simulink model "model_VS_PSH"  (R2020b)
settings: Solver=ode1  StartTime=0.0  StopTime=60  RelTol=1e-3
InitFcn:
  | xInitial = init_power_wind_dfig_det;
  | %Ts=5e-6;
values from neighbouring files (symbols this model uses):
  Cap_DClink = 20000e-6    (= 0.02)    [MAIN_VS_PSH.m]
  Efficiency = 0.9    [MAIN_VS_PSH.m]
  Fnom = 60    [MAIN_VS_PSH.m]
  H = 2.7    [MAIN_VS_PSH.m]
  Initial_Head = 1    [MAIN_VS_PSH.m]
  Initial_SOC = 0.8    [MAIN_VS_PSH.m]
  kmVdc = 20e3    (= 20000)    [MAIN_VS_PSH.m]
  Kp = 1    [MAIN_VS_PSH.m]
  kp_pll = 0.236583    [MAIN_T_PSH_IEEE39.m]    (also in MAIN_VS_PSH.m)
  Kpg = 1.3466e-5    (= 1.3466e-05)    [MAIN_VS_PSH.m]
  Kpr = 4.559e-5    (= 4.559e-05)    [MAIN_VS_PSH.m]
  Kvp = 6.1584    [MAIN_VS_PSH.m]
  Lm = Lb*Lmpu    [MAIN_VS_PSH.m]
  Lph = 3e-4    (= 0.0003)    [MAIN_VS_PSH.m]
  Lr = Lb*Lrpu    [MAIN_VS_PSH.m]
  Lrleakpu = 0.11    [MAIN_VS_PSH.m]
  Ls = Lb*Lspu    [MAIN_VS_PSH.m]
  Lsleakpu = 0.102    [MAIN_VS_PSH.m]
  Max_discharge_hrs = 10    [MAIN_VS_PSH.m]
  Mode = 0    [MAIN_FS_PSH_IEEE39.m]    (also in MAIN_VS_PSH.m = 1; plots_FS_PSH_IEEE39.m = 1; plots_VS_PSH.m = 1)
  Pnom = Srated*1e6    (= 300000000)    [MAIN_VS_PSH.m]
  Pref = 0.9    [MAIN_T_PSH_IEEE39.m]    (also in MAIN_VS_PSH.m = 1)
  QnL = 0    [MAIN_VS_PSH.m]
  Qref = 0    [MAIN_VS_PSH.m]
  Rrpu = 0.00607    [MAIN_VS_PSH.m]
  Rspu = 0.0054    [MAIN_VS_PSH.m]
  sigma = 1- Lmpu*Lmpu/(Lrpu^2)    (= 0.0485899542692)    [MAIN_VS_PSH.m]
  Srated = 300    [MAIN_VS_PSH.m]
  t_sw_off = 220    [MAIN_FS_PSH_IEEE39.m]    (also in MAIN_T_PSH_IEEE39.m; MAIN_VS_PSH.m = 45)
  t_sw_on = 130    [MAIN_FS_PSH_IEEE39.m]    (also in MAIN_T_PSH_IEEE39.m; MAIN_VS_PSH.m = 35)
  Ti = 0.01    [MAIN_VS_PSH.m]
  ti_pll = 0.0224242    [MAIN_T_PSH_IEEE39.m]    (also in MAIN_VS_PSH.m)
  Tig = 59.0944    [MAIN_VS_PSH.m]
  Tir = 197.953    [MAIN_VS_PSH.m]
  Ts = 25e-6    (= 2.5e-05)    [MAIN_FS_PSH_IEEE39.m]    (also in MAIN_T_PSH_IEEE39.m; MAIN_VS_PSH.m = 1e-07)
  TurnsRatio = 0.37912    [MAIN_VS_PSH.m]
  Tvi = 0.0013532    [MAIN_VS_PSH.m]
  V1 = sqrt(2)*Vnom_grid/sqrt(3)    [MAIN_VS_PSH.m]
  Vdc_ref = 40e3    (= 40000)    [MAIN_VS_PSH.m]
  Vnom_grid = 18e3    (= 18000)    [MAIN_VS_PSH.m]
  W1 = 2*pi*Fnom    (= 376.991118431)    [MAIN_VS_PSH.m]
  Xph = Lph*W1    (= 0.113097335529)    [MAIN_VS_PSH.m]
undefined symbols (not defined in the file or in its folder): magnitude
libraries: powerlib x49, powerlib_meascontrol x21, pid_lib x10, simulink_extras x4, simulink x1
(part 3 of 3)

== system model_VS_PSH/Subsystem2/Subsystem5/Measurement and Transformation/Subsystem ==
  Vabc : Inport
  Constant : Constant  Value=2*pi*60
  Demux : Demux  Outputs=3
  Gain : Gain  Gain=1/(2*pi)
  Integrator : Integrator
  MATLAB Function1 : MATLAB Function  TreatAsAtomicUnit=on
  PID Controller : pid_lib/PID Controller  Controller=PI  Form=Parallel  TimeDomain=Continuous-time  UseExternalTs=off  SampleTime=-1  IntegratorMethod=Forward Euler  FilterMethod=Forward Euler  ControllerParametersSource=internal  P=kp_pll  I=kp_pll/ti_pll  D=0  UseFilter=on  N=100  TunerSelectOption=Transfer Function Based (PID Tuner App)  InitialConditionSource=internal  InitialConditionForIntegrator=0  InitialConditionForFilter=0  DifferentiatorICPrevScaledInput=0  ExternalReset=none  TrackingMode=off  Kt=1  LimitOutput=off  SatLimitsSource=internal  UpperSaturationLimit=inf  LowerSaturationLimit=-inf  LinearizeAsGain=on  AntiWindupMode=none  Kb=1  POutMin=[]  POutMax=[]  IOutMin=[]  IOutMax=[]  DOutMin=[]  DOutMax=[]  NOutMin=[]  NOutMax=[]  SumOutMin=[]  SumOutMax=[]  SaturationOutMin=[]  SaturationOutMax=[]  PParamMin=[]  PParamMax=[]  IParamMin=[]  IParamMax=[]  DParamMin=[]  DParamMax=[]  NParamMin=[]  NParamMax=[]  KbParamMin=[]  KbParamMax=[]  KtParamMin=[]  KtParamMax=[]  KbOutMin=[]  KbOutMax=[]  KtOutMin=[]  KtOutMax=[]  IntegratorOutMin=[]  IntegratorOutMax=[]  FilterOutMin=[]  FilterOutMax=[]  SumI1OutMin=[]  SumI1OutMax=[]  SumI2OutMin=[]  SumI2OutMax=[]  SumI3OutMin=[]  SumI3OutMax=[]  SumI4OutMin=[]  SumI4OutMax=[]  SumDOutMin=[]  SumDOutMax=[]  DifferentiatorOutMin=[]  DifferentiatorOutMax=[]  FilterDiffOutCoefMin=[]  FilterDiffOutCoefMax=[]  ReciprocalOutMin=[]  ReciprocalOutMax=[]  SumDenOutMin=[]  SumDenOutMax=[]  SumNumOutMin=[]  SumNumOutMax=[]  DivideOutMin=[]  DivideOutMax=[]  UdiffTsProdOutMin=[]  UdiffTsProdOutMax=[]  NTsProdOutMin=[]  NTsProdOutMax=[]  UintegralTsProdOutMin=[]  UintegralTsProdOutMax=[]  UngainTsProdOutMin=[]  UngainTsProdOutMax=[]  IntegratorContinuousStateAttributes=''  IntegratorStateMustResolveToSignalObject=off  IntegratorRTWStateStorageClass=Auto  FilterContinuousStateAttributes=''  FilterStateMustResolveToSignalObject=off  FilterRTWStateStorageClass=Auto  ParallelPVariant=InternalParameters  IdealPVariant=Disabled  IVariant=InternalParameters  DVariant=Disabled  IntegratorVariant=Continuous  SatVariant=Disabled  AWVariant=Passthrough  PCopyVariant=Disabled  TRVariant=Disabled  FdbkBlocksVariant=Forward  IdealPFdbkVariant=Disabled  SatFdbkVariant=Disabled  DerivativeFilterVariant=Disabled  NVariant=Disabled  NCopyVariant=Disabled_SignalSpec  FilterICVariant=Disabled  IntegratorICVariant=InternalICs  ExternalResetVariant=Disabled  TRSumVariant=Passthrough  SumFdbkVariant=Disabled  SumVariant=Sum_PI  TsampFilterVariant=InternalTs  TsampNgainVariant=Passthrough  TsampIntegralVariant=Passthrough  ExternalSaturationOutDataTypeStr=Inherit: Same as second input
  Scope2 : Scope
  Sum5 : Sum  Inputs=|++
  Terminator : Terminator
  Terminator1 : Terminator
  abc to dq0 : powerlib_meascontrol/Transformations/abc to dq0  Alignment=Aligned with phase A axis
  angle : Outport
  Freq_Hz : Outport  Port=2
  wires:
  Constant/1 -> Sum5/2
  PID Controller/1 -> Sum5/1
  Vabc/1 -> abc to dq0/1
  Demux/3 -> Terminator/1
  Demux/1 -> Terminator1/1
  Demux/2 -> PID Controller/1
  Sum5/1 -> Gain/1, Integrator/1
  Integrator/1 -> Scope2/1, MATLAB Function1/1(u)
  Gain/1 -> Freq_Hz/1
  MATLAB Function1/1(y) -> abc to dq0/2, angle/1
  abc to dq0/1 -> Demux/1

== system model_VS_PSH/Subsystem2/Subsystem5/Rotor-side Controls/Subsystem1 ==
  In : Inport
  Gain1 : Gain  Gain=1/Ti
  Gain2 : Gain  Gain=Kp
  Gain3 : Gain
  Integrator : Integrator
  Saturation : Saturate  UpperLimit=100e3  LowerLimit=-100e3
  Sum2 : Sum  Inputs=|++
  Sum3 : Sum  Inputs=-+|
  Sum7 : Sum  Inputs=|++
  Out : Outport
  wires:
  In/1 -> Sum7/1, Gain2/1
  Saturation/1 -> Sum3/2, Out/1
  Gain2/1 -> Sum2/1
  Sum2/1 -> Sum3/1, Saturation/1
  Sum3/1 -> Gain3/1
  Gain1/1 -> Integrator/1
  Integrator/1 -> Sum2/2
  Gain3/1 -> Sum7/2
  Sum7/1 -> Gain1/1

== system model_VS_PSH/Subsystem2/Subsystem5/Rotor-side Controls/Subsystem2 ==
  In : Inport
  Gain1 : Gain  Gain=1/Ti
  Gain2 : Gain  Gain=Kp
  Gain3 : Gain
  Integrator : Integrator
  Saturation : Saturate  UpperLimit=100e3  LowerLimit=-100e3
  Sum2 : Sum  Inputs=|++
  Sum3 : Sum  Inputs=-+|
  Sum7 : Sum  Inputs=|++
  Out : Outport
  wires:
  In/1 -> Sum7/1, Gain2/1
  Saturation/1 -> Sum3/2, Out/1
  Gain2/1 -> Sum2/1
  Sum2/1 -> Sum3/1, Saturation/1
  Sum3/1 -> Gain3/1
  Gain1/1 -> Integrator/1
  Integrator/1 -> Sum2/2
  Gain3/1 -> Sum7/2
  Sum7/1 -> Gain1/1

== system model_VS_PSH/Subsystem2/Subsystem5/Rotor-side Controls/Subsystem3 ==
  In : Inport
  Gain1 : Gain  Gain=1/Ti
  Gain2 : Gain  Gain=Kp
  Gain3 : Gain
  Integrator : Integrator
  Saturation : Saturate  UpperLimit=100e3  LowerLimit=-100e3
  Sum2 : Sum  Inputs=|++
  Sum3 : Sum  Inputs=-+|
  Sum7 : Sum  Inputs=|++
  Out : Outport
  wires:
  In/1 -> Sum7/1, Gain2/1
  Saturation/1 -> Sum3/2, Out/1
  Gain2/1 -> Sum2/1
  Sum2/1 -> Sum3/1, Saturation/1
  Sum3/1 -> Gain3/1
  Gain1/1 -> Integrator/1
  Integrator/1 -> Sum2/2
  Gain3/1 -> Sum7/2
  Sum7/1 -> Gain1/1

== system model_VS_PSH/Subsystem2/Subsystem5/Rotor-side Controls/Subsystem4 ==
  In : Inport
  Gain1 : Gain  Gain=1/Ti
  Gain2 : Gain  Gain=Kp
  Gain3 : Gain
  Integrator : Integrator
  Saturation : Saturate  UpperLimit=100e3  LowerLimit=-100e3
  Sum2 : Sum  Inputs=|++
  Sum3 : Sum  Inputs=-+|
  Sum7 : Sum  Inputs=|++
  Out : Outport
  wires:
  In/1 -> Sum7/1, Gain2/1
  Saturation/1 -> Sum3/2, Out/1
  Gain2/1 -> Sum2/1
  Sum2/1 -> Sum3/1, Saturation/1
  Sum3/1 -> Gain3/1
  Gain1/1 -> Integrator/1
  Integrator/1 -> Sum2/2
  Gain3/1 -> Sum7/2
  Sum7/1 -> Gain1/1

== matlab function model_VS_PSH/Subsystem2/Subsystem5/Measurement and Transformation/MATLAB Function2 ==
  data: u input; y output
function y = fcn(u)



if u>= 2*pi
    y = mod(u,2*pi);
elseif u <= 0
    y = 2*pi - mod(abs(u),2*pi);
else
    y = u;
end

== matlab function model_VS_PSH/Subsystem2/Subsystem5/Measurement and Transformation/Subsystem/MATLAB Function1 ==
  data: u input; y output
function y = fcn(u)



if u>= 2*pi
    y = mod(u,2*pi);
elseif u <= 0
    y = 2*pi - mod(abs(u),2*pi);
else
    y = u;
end

== matlab function model_VS_PSH/Subsystem2/Subsystem5/Measurement and Transformation/MATLAB Function1 ==
  data: u input; y output
function y = fcn(u)



if u>= 2*pi
    y = mod(u,2*pi);
elseif u <= 0
    y = 2*pi - mod(abs(u),2*pi);
else
    y = u;
end
